simulink model "robot3_no_model_slidingmode_control"  (R2023b)
settings: Solver=FixedStepAuto  StartTime=0.0  StopTime=4*pi  RelTol=1e-3
undefined symbols (not defined in the file or in its folder): Cartesian_trajectory, Coriolis3, Dinv3, Forward_kin3, Gravity3
libraries: simulink x1
settings Model: Creator=사용자  LastModifiedBy=Chan
settings SolverCC: ZeroCrossAlgorithm=Adaptive
settings DebuggingCC: IgnoredZcDiagnostic=none

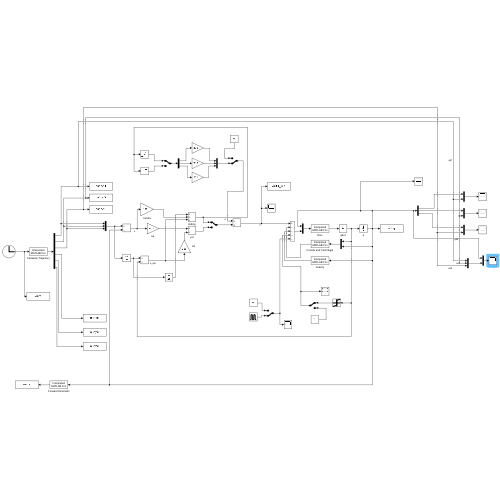
[thumbnail: Simulink's stored preview of the top-level diagram]
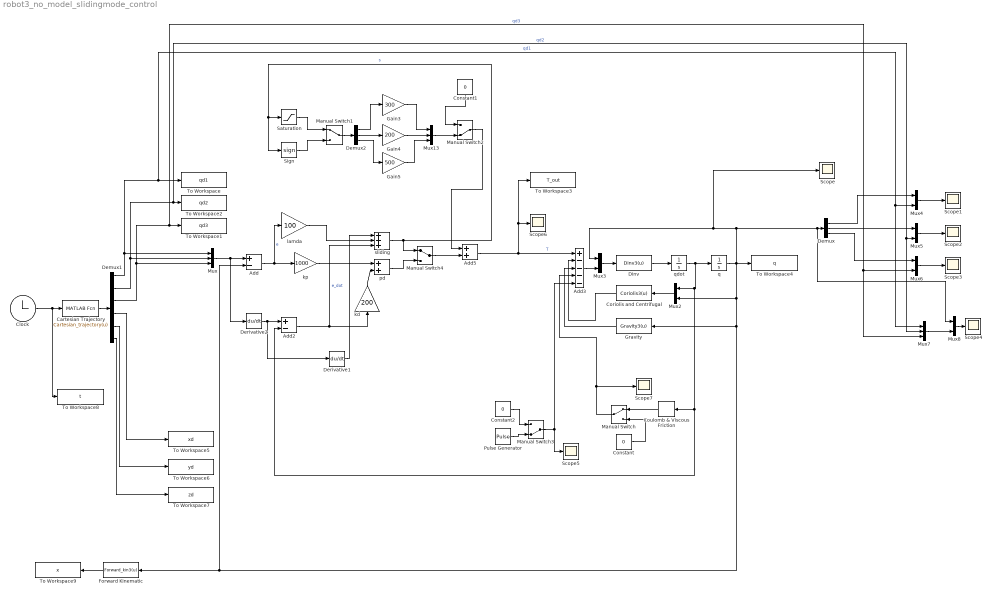
== system robot3_no_model_slidingmode_control ==
  Add : Sum  Inputs=+-
  Add2 : Sum  Inputs=+-
  Add3 : Sum  Inputs=+----
  Add5 : Sum
  Cartesian Trajectory : MATLABFcn  MATLABFcn=Cartesian_trajectory(u)  OutputDimensions=6  Output1D=off
  Clock : Clock
  Constant : Constant  Value=0
  Constant1 : Constant  Value=0
  Constant2 : Constant  Value=0
  Coriolis and Centrifugal : MATLABFcn  MATLABFcn=Coriolis3(u)  OutputDimensions=3  Output1D=off
  Coulomb & Viscous Friction : simulink/Discontinuities/Coulomb & Viscous Friction  offset=10  gain=5
  Demux : Demux  Outputs=3
  Demux1 : Demux  Outputs=6
  Demux2 : Demux  Outputs=3
  Derivative1 : Derivative  CoefficientInTFapproximation=1000
  Derivative2 : Derivative  CoefficientInTFapproximation=1000
  Dinv : MATLABFcn  MATLABFcn=Dinv3(u)  OutputDimensions=3  Output1D=off
  Forward Kinematic : MATLABFcn  MATLABFcn=Forward_kin3(u)  OutputDimensions=3  Output1D=off
  Gain3 : Gain  Gain=300
  Gain4 : Gain  Gain=200
  Gain5 : Gain  Gain=500
  Gravity : MATLABFcn  MATLABFcn=Gravity3(u)  OutputDimensions=3  Output1D=off
  Manual Switch : ManualSwitch
  Manual Switch1 : ManualSwitch
  Manual Switch2 : ManualSwitch  CurrentSetting=0
  Manual Switch3 : ManualSwitch  CurrentSetting=0
  Manual Switch4 : ManualSwitch
  Mux : Mux  Inputs=3
  Mux13 : Mux  Inputs=3
  Mux{2..6,8} (6 alike) : Mux  Inputs=2
  Mux7 : Mux  Inputs=3
  Pulse Generator : DiscretePulseGenerator  PulseType=Time based  Amplitude=100  Period=0.2  PulseWidth=2  PhaseDelay=2
  Saturation : Saturate  UpperLimit=1  LowerLimit=-1
  Scope{,1..7} (8 alike) : Scope
  Sign : Signum
  To Workspace : ToWorkspace  VariableName=qd1  SaveFormat=Timeseries  SampleTime=0.001
  To Workspace1 : ToWorkspace  VariableName=qd3  SaveFormat=Timeseries  SampleTime=0.001
  To Workspace2 : ToWorkspace  VariableName=qd2  SaveFormat=Timeseries  SampleTime=0.001
  To Workspace3 : ToWorkspace  VariableName=T_out  SampleTime=0.001
  To Workspace4 : ToWorkspace  VariableName=q  SaveFormat=Timeseries  SampleTime=0.001
  To Workspace5 : ToWorkspace  VariableName=xd  SampleTime=0.001
  To Workspace6 : ToWorkspace  VariableName=yd  SampleTime=0.001
  To Workspace7 : ToWorkspace  VariableName=zd  SampleTime=0.001
  To Workspace8 : ToWorkspace  VariableName=t  SaveFormat=Timeseries  SampleTime=0.001
  To Workspace9 : ToWorkspace  VariableName=x  SampleTime=0.001
  kd : Gain  Gain=200
  kp : Gain  Gain=1000
  lamda : Gain  Gain=100
  pd : Sum
  q : Integrator  InitialCondition=[0.9587;0.7246;-1.1694]
  qdot : Integrator  InitialCondition=[0;0;0];
  sliding : Sum  Inputs=+++
  wires:
  kp/1 -> pd/1
  kd/1 -> pd/2
  Add3/1 -> Mux3/2
  Mux3/1 -> Dinv/1
  Dinv/1 -> qdot/1
  Mux2/1 -> Coriolis and Centrifugal/1
  qdot/1 -> Add2/2, Coulomb & Viscous Friction/1, Mux2/1, q/1
  Coriolis and Centrifugal/1 -> Add3/2
  Gravity/1 -> Add3/3
  q/1 -> Mux8/1, Demux/1, Scope/1, Mux3/1, To Workspace4/1, Forward Kinematic/1, Add/2, Gravity/1, Mux2/2
  Mux4/1 -> Scope1/1
  Mux5/1 -> Scope2/1
  Mux6/1 -> Scope3/1
  Demux/1 -> Mux4/1
  Demux/2 -> Mux5/1
  Demux/3 -> Mux6/1
  Mux7/1 -> Mux8/2
  Mux8/1 -> Scope4/1
  Cartesian Trajectory/1 -> Demux1/1
  Demux1/1 -> Mux/1, To Workspace/1, Mux7/1, Mux4/2  "qd1"
  Demux1/2 -> Mux/2, Mux7/2, Mux5/2, To Workspace2/1  "qd2"
  Demux1/3 -> Mux/3, To Workspace1/1, Mux7/3, Mux6/2  "qd3"
  Demux1/4 -> To Workspace5/1
  Demux1/5 -> To Workspace6/1
  Demux1/6 -> To Workspace7/1
  Mux/1 -> Add/1, Derivative2/1
  Clock/1 -> To Workspace8/1, Cartesian Trajectory/1
  Forward Kinematic/1 -> To Workspace9/1
  Coulomb & Viscous Friction/1 -> Manual Switch/1
  Constant/1 -> Manual Switch/2
  Manual Switch/1 -> Scope7/1, Add3/4
  Manual Switch1/1 -> Demux2/1
  Saturation/1 -> Manual Switch1/1
  Sign/1 -> Manual Switch1/2
  Demux2/1 -> Gain3/1
  Demux2/2 -> Gain4/1
  Gain3/1 -> Mux13/1
  Gain4/1 -> Mux13/2
  Gain5/1 -> Mux13/3
  Demux2/3 -> Gain5/1
  Mux13/1 -> Manual Switch2/2
  Constant1/1 -> Manual Switch2/1
  Constant2/1 -> Manual Switch3/1
  Manual Switch3/1 -> Scope5/1, Add3/5
  Pulse Generator/1 -> Manual Switch3/2
  Add5/1 -> Add3/1, To Workspace3/1, Scope6/1  "T"
  Derivative2/1 -> Add2/1, Derivative1/1
  Add2/1 -> kd/1, sliding/3  "e_dot"
  Add/1 -> lamda/1, kp/1  "e"
  sliding/1 -> Sign/1, Saturation/1, Manual Switch4/1  "s"
  pd/1 -> Manual Switch4/2
  Manual Switch4/1 -> Add5/2
  Manual Switch2/1 -> Add5/1
  Derivative1/1 -> sliding/1
  lamda/1 -> sliding/2
